simulink model "ElectricalScheme"  (R2025b)
settings: Solver=VariableStepAuto  StartTime=0.0  StopTime=10  RelTol=1e-6
model workspace (MAT data in the model file):
  B = 0.1
  D = 0.4
  J = 0.01
  Ke = 0.01
  Kt = 0.01
  L = 0.5
  Req = 1
  Vbat = 24
settings Model: Creator=khalid  LastModifiedBy=khalid

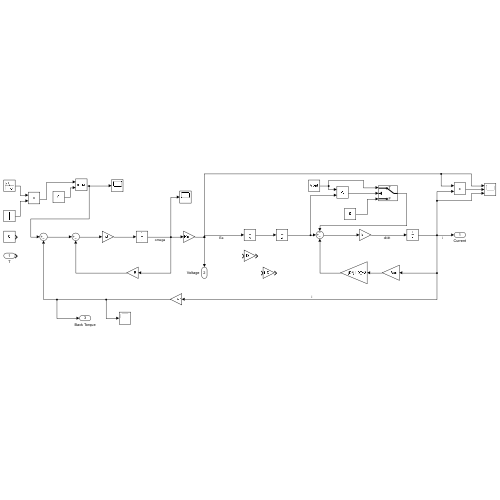
[thumbnail: Simulink's stored preview of the top-level diagram]
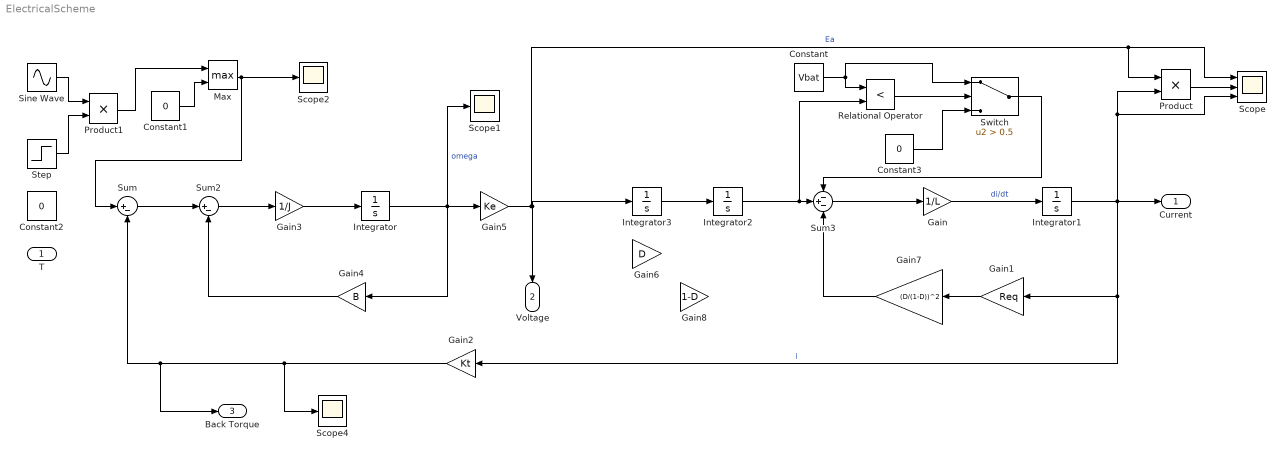
== system ElectricalScheme ==
  T : Inport
  Constant : Constant  Value=Vbat
  Constant1 : Constant  Value=0
  Constant2 : Constant  Value=0
  Constant3 : Constant  Value=0
  Gain : Gain  Gain=1/L
  Gain1 : Gain  Gain=Req
  Gain2 : Gain  Gain=Kt
  Gain3 : Gain  Gain=1/J
  Gain4 : Gain  Gain=B
  Gain5 : Gain  Gain=Ke
  Gain6 : Gain  Gain=D
  Gain7 : Gain  Gain=(D/(1-D))^2
  Gain8 : Gain  Gain=1-D
  Integrator{,1..3} (4 alike) : Integrator
  Max : MinMax  Function=max  Inputs=2
  Product : Product
  Product1 : Product
  Relational Operator : RelationalOperator  Operator=<  OutDataTypeStr=boolean  RndMeth=Simplest  InputSameDT=off
  Scope : Scope  NumInputPorts=3
      settings: ActiveDisplayYMinimum=-7.2605692447526673  ActiveDisplayYMaximum=64.818299057419381
  Scope1 : Scope
      settings: ActiveDisplayYMinimum=-729.29894  ActiveDisplayYMaximum=6560.77635
  Scope2 : Scope
      settings: ActiveDisplayYMinimum=-124.9931  ActiveDisplayYMaximum=1124.93794  DataLoggingVariableName=ScopeData2
  Scope4 : Scope
      settings: ActiveDisplayYMinimum=-0.26973  ActiveDisplayYMaximum=0.02997  DataLoggingVariableName=ScopeData4
  Sine Wave : Sin  Amplitude=1e3  Frequency=20  SampleTime=0
  Step : Step  Time=5  Before=1  After=0  SampleTime=0
  Sum : Sum  Inputs=|+-
  Sum2 : Sum  Inputs=|+-
  Sum3 : Sum  Inputs=-+-
  Switch : Switch  Criteria=u2 > Threshold  Threshold=0.5  SaturateOnIntegerOverflow=off  InputSameDT=off
  Current : Outport
  Voltage : Outport  Port=2
  Back Torque : Outport  Port=3
  wires:
  Gain4/1 -> Sum2/2
  Gain3/1 -> Integrator/1
  Integrator/1 -> Gain5/1, Gain4/1, Scope1/1  "omega"
  Gain2/1 -> Scope4/1, Back Torque/1, Sum/2
  Integrator1/1 -> Gain1/1, Gain2/1, Current/1, Product/2, Scope/3  "i"
  Sum/1 -> Sum2/1
  Gain5/1 -> Integrator3/1, Voltage/1, Product/1, Scope/1  "Ea"
  Gain/1 -> Integrator1/1  "di/dt"
  Sum2/1 -> Gain3/1
  Product/1 -> Scope/2
  Sine Wave/1 -> Product1/1
  Step/1 -> Product1/2
  Constant1/1 -> Max/2
  Product1/1 -> Max/1
  Max/1 -> Sum/1, Scope2/1
  Gain1/1 -> Gain7/1
  Sum3/1 -> Gain/1
  Constant/1 -> Switch/1, Relational Operator/1
  Constant3/1 -> Switch/3
  Switch/1 -> Sum3/1
  Relational Operator/1 -> Switch/2
  Integrator2/1 -> Sum3/2, Relational Operator/2
  Gain7/1 -> Sum3/3
  Integrator3/1 -> Integrator2/1
